simulink model "washing_machine"  (R2024b)
settings: Solver=VariableStepAuto  StartTime=0.0  StopTime=inf  RelTol=1e-3
settings Model: Creator=DELL  LastModifiedBy=DELL

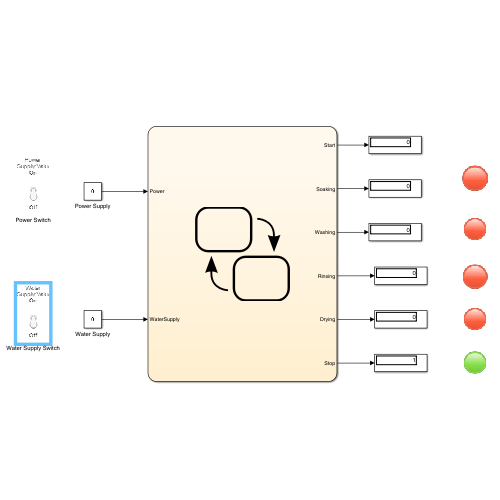
[thumbnail: Simulink's stored preview of the top-level diagram]
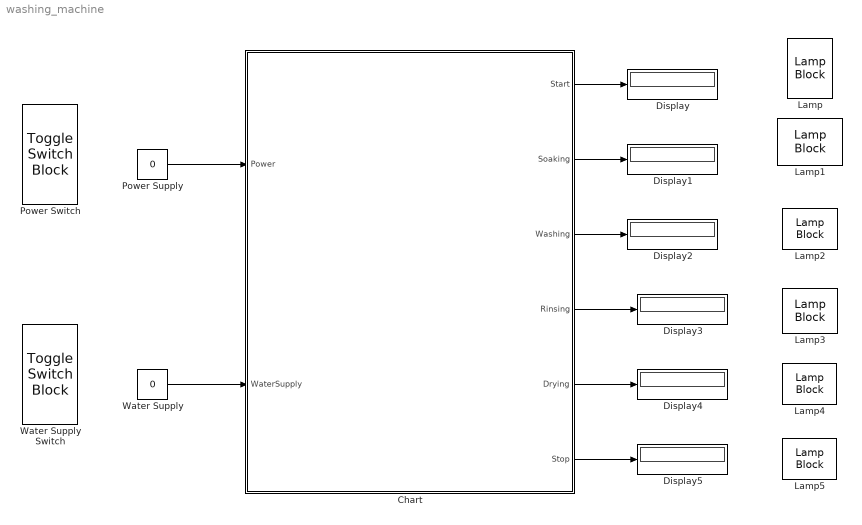
== system washing_machine ==
  Chart : Stateflow chart  TreatAsAtomicUnit=on
  Display{,1..5} (6 alike) : Display
  Lamp{,1..5} (6 alike) : LampBlock  LabelPosition=Hide
  Power Supply : Constant  Value=0
  Power Switch : ToggleSwitchBlock
      settings: Values={{'Off', 'On'}, [0 1]}
  Water Supply : Constant  Value=0
  Water Supply Switch : ToggleSwitchBlock
      settings: Values={{'Off', 'On'}, [0 1]}
  wires:
  Chart/1(Start) -> Display/1
  Chart/2(Soaking) -> Display1/1
  Chart/3(Washing) -> Display2/1
  Chart/4(Rinsing) -> Display3/1
  Chart/5(Drying) -> Display4/1
  Chart/6(Stop) -> Display5/1
  Power Supply/1 -> Chart/1(Power)
  Water Supply/1 -> Chart/2(WaterSupply)

== stateflow chart washing_machine/Chart ==
  state Power
  state ON
    entry:Start=1
  state Water_Supply
  state Soaking
    entry:Soaking=1
  state Washing
    entry:Washing=1
  state Rinsing
    entry:Rinsing=1
  state Drying
    entry:Drying=1
  state OFF
    entry:Stop=1
  (default) -> Power
  Power -> (junction 18) [order 2] : [Power==0]
  Power -> ON [order 1] : [Power==1]
  ON -> Water_Supply
  (junction 18) -> (junction 17)
  Water_Supply -> (junction 17) [order 2] : [WaterSupply==0]
  Water_Supply -> Soaking [order 1] : [WaterSupply==1]
  Soaking -> Washing : [after(200,sec)]
  Washing -> Rinsing : [after(100,sec)]
  (junction 17) -> OFF
  Rinsing -> Drying : [after(20,sec)]
  Drying -> OFF : [after(50,sec)]
  data: Power input; WaterSupply input; Start output; Soaking output; Washing output; Rinsing output; Drying output; Stop output
